simulink model "test_integrator"  (R2026a)
settings: Solver=VariableStepAuto  StopTime=20
undefined symbols (not defined in the file): m, P
settings Model: Creator=User  LastModifiedBy=Kiril

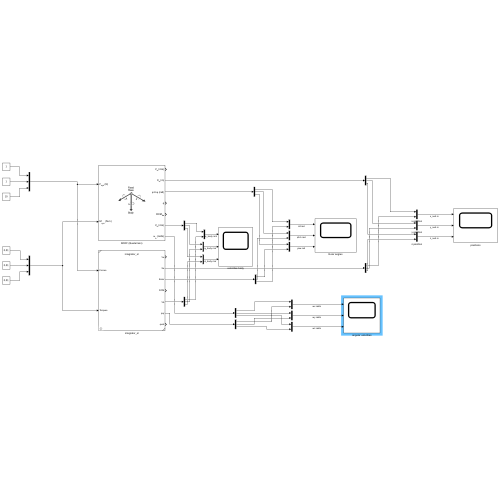
[thumbnail: Simulink's stored preview of the top-level diagram]
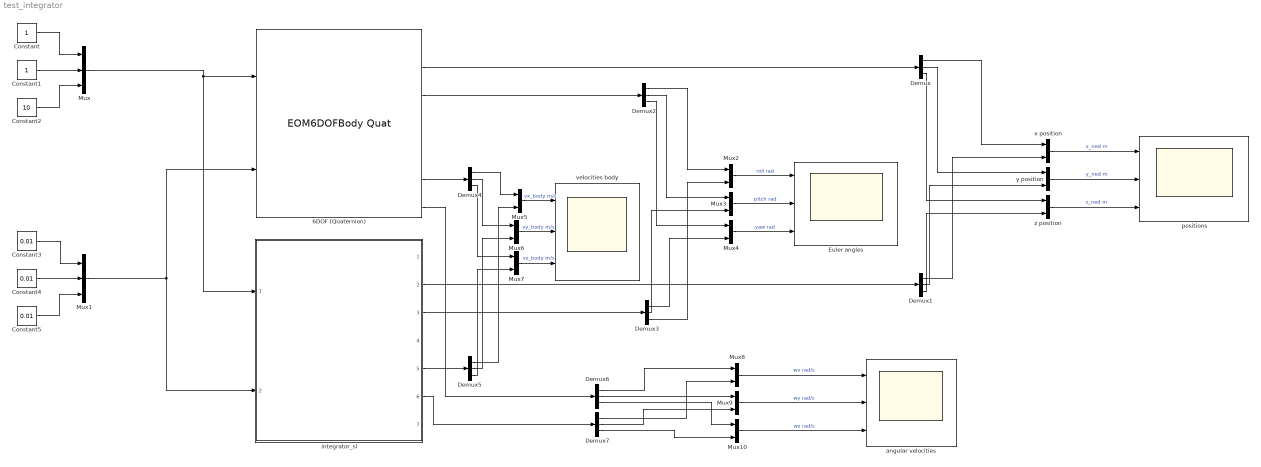
== system test_integrator ==
  6DOF (Quaternion) : EOM6DOFBodyQuat  xme_0=Sim.Initial_Position  Vm_0=Sim.Initial_Velocity_Body  eul_0=Sim.Initial_Euler_Angles_Rad  pm_0=Sim.Initial_Body_Angular_Rates_Rads  mass_0=m  inertia=P.I
  Constant : Constant
  Constant1 : Constant
  Constant2 : Constant  Value=10
  Constant3 : Constant  Value=0.01
  Constant4 : Constant  Value=0.01
  Constant5 : Constant  Value=0.01
  Demux{,1..7} (8 alike) : Demux  Outputs=3
  Euler angles : Scope  NumInputPorts=3
      settings: ActiveDisplayYMinimum=-1.9203839226792738  ActiveDisplayYMaximum=2.5904237640219541
  Mux : Mux  Inputs=3
  Mux1 : Mux  Inputs=3
  Mux{2..10} (9 alike) : Mux  Inputs=2
  angular velocities : Scope  NumInputPorts=3
      settings: ActiveDisplayYMinimum=-4.4540793653359918  ActiveDisplayYMaximum=3.6016943028276502  DataLoggingVariableName=ScopeData3
  integrator_sl : Subsystem  ReferencedSubsystem=integrator_sl  Mass=m  Inertia=P.I  Pos=Sim.Initial_Position  Velocity=Sim.Initial_Velocity_Body  Orient=Sim.Initial_Euler_Angles_Rad  AngVelocity=Sim.Initial_Body_Angular_Rates_Rads
  positions : Scope  NumInputPorts=3
      settings: ActiveDisplayYMinimum=-91.23651647450383  ActiveDisplayYMaximum=821.12864827053454
  velocities body : Scope  NumInputPorts=3
      settings: ActiveDisplayYMinimum=-27.805911392749895  ActiveDisplayYMaximum=26.304735635570225  DataLoggingVariableName=ScopeData2
  x position : Mux  Inputs=2
  y position : Mux  Inputs=2
  z position : Mux  Inputs=2
  wires:
  Mux1/1 -> 6DOF (Quaternion)/2, integrator_sl/2
  Mux/1 -> integrator_sl/1, 6DOF (Quaternion)/1
  Constant/1 -> Mux/1
  Constant1/1 -> Mux/2
  Constant2/1 -> Mux/3
  Constant3/1 -> Mux1/1
  Constant4/1 -> Mux1/2
  Constant5/1 -> Mux1/3
  6DOF (Quaternion)/2 -> Demux/1
  integrator_sl/2 -> Demux1/1
  Demux/1 -> x position/1
  Demux1/1 -> x position/2
  Demux/2 -> y position/1
  Demux1/2 -> y position/2
  Demux/3 -> z position/1
  Demux1/3 -> z position/2
  x position/1 -> positions/1  "x_ned m"
  y position/1 -> positions/2  "y_ned m"
  z position/1 -> positions/3  "z_ned m"
  6DOF (Quaternion)/3 -> Demux2/1
  integrator_sl/3 -> Demux3/1
  Demux2/1 -> Mux2/1
  Demux3/3 -> Mux2/2
  Demux2/2 -> Mux3/1
  Demux2/3 -> Mux4/1
  Demux3/2 -> Mux3/2
  Demux3/1 -> Mux4/2
  Mux2/1 -> Euler angles/1  "roll rad"
  Mux3/1 -> Euler angles/2  "pitch rad"
  Mux4/1 -> Euler angles/3  "yaw rad"
  6DOF (Quaternion)/6 -> Demux4/1
  integrator_sl/5 -> Demux5/1
  Demux4/1 -> Mux5/1
  Demux5/1 -> Mux5/2
  Demux4/2 -> Mux6/1
  Demux5/2 -> Mux6/2
  Demux4/3 -> Mux7/1
  Demux5/3 -> Mux7/2
  Mux5/1 -> velocities body/1  "vx_body m/s"
  Mux6/1 -> velocities body/2  "vy_body m/s"
  Mux7/1 -> velocities body/3  "vz_body m/s"
  6DOF (Quaternion)/7 -> Demux6/1
  integrator_sl/6 -> Demux7/1
  Demux6/1 -> Mux8/1
  Demux7/1 -> Mux8/2
  Demux6/2 -> Mux9/1
  Demux7/2 -> Mux9/2
  Demux6/3 -> Mux10/1
  Demux7/3 -> Mux10/2
  Mux8/1 -> angular velocities/1  "wx rad/s"
  Mux9/1 -> angular velocities/2  "wy rad/s"
  Mux10/1 -> angular velocities/3  "wz rad/s"
